simulink model "Aircraft_Model"  (R2026a)
settings: Solver=VariableStepAuto  StopTime=tEnd
values from neighbouring files (symbols this model uses):
  tEnd = 75    [Initial_Conds.m]
  U0 = [delta_ail;delta_ele;delta_rud;delta_thr]    [Initial_Conds.m]
  x0 = [x0;y0;z0;u0;v0;w0;phi0;theta0;psi0;p0;q0;r0]    [Initial_Conds.m]
undefined symbols (not defined in the file or in its folder): Non_Linear_Model_V1
libraries: aerolibanim x1
settings Model: Creator=hakka  LastModifiedBy=hakka

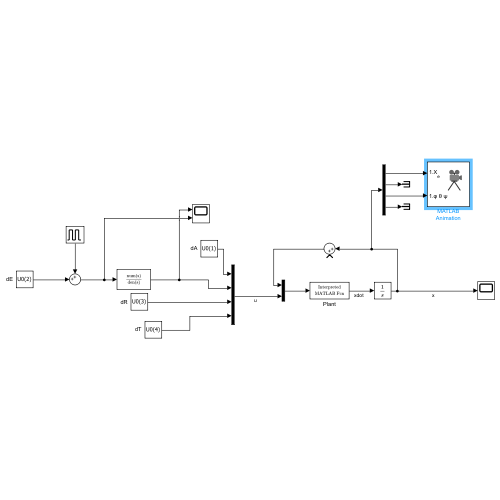
[thumbnail: Simulink's stored preview of the top-level diagram]
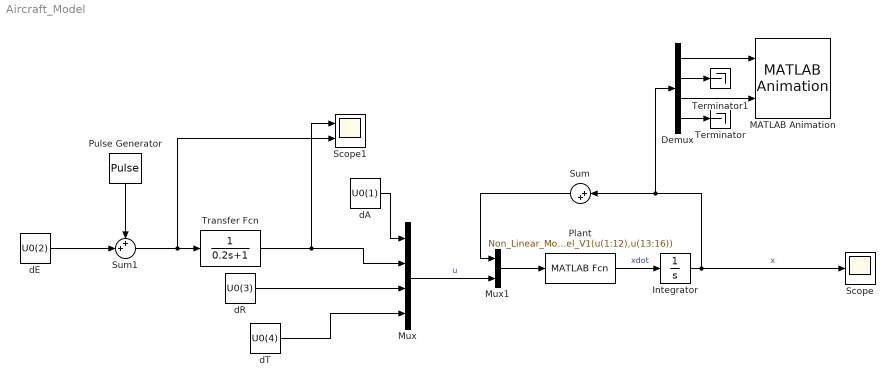
== system Aircraft_Model ==
  Demux : Demux  Outputs=[3 3 3 3]
  Integrator : Integrator  InitialCondition=x0
  MATLAB Animation : aerolibanim/MATLAB Animation  Tag=Matlab Animation 6 DOF  Vehicles=1  Geometries='pa24-250_orange.ac'  BoundingBoxCoordinates=[-100,100,-100,100,-100,100]  CameraOffset=[150,150,0]  CameraViewAngle=3  SampleTime=0.1  FigurePosition=[403,50,619,758]
  Mux : Mux
  Mux1 : Mux  Inputs=2
  Plant : MATLABFcn  MATLABFcn=Non_Linear_Model_V1(u(1:12),u(13:16))
  Pulse Generator : DiscretePulseGenerator  PulseType=Time based  Amplitude=0.05  Period=(tEnd/2)+5  PulseWidth=5  PhaseDelay=25
  Scope : Scope
      settings: ActiveDisplayYMinimum=-0.21358140820806887  ActiveDisplayYMaximum=0.10465761191012857
  Scope1 : Scope  NumInputPorts=2
      settings: ActiveDisplayYMinimum=-0.014196127760530999  ActiveDisplayYMaximum=0.048303872239469005
  Sum : Sum  Inputs=|++
  Sum1 : Sum  Inputs=++|
  Terminator : Terminator
  Terminator1 : Terminator
  Transfer Fcn : TransferFcn  Numerator=1  Denominator=[0.2 1]
  dA : Constant  Value=U0(1)
  dE : Constant  Value=U0(2)
  dR : Constant  Value=U0(3)
  dT : Constant  Value=U0(4)
  wires:
  Plant/1 -> Integrator/1  "xdot"
  Integrator/1 -> Scope/1, Demux/1, Sum/1  "x"
  dA/1 -> Mux/1
  dR/1 -> Mux/3
  dT/1 -> Mux/4
  Mux/1 -> Mux1/2  "u"
  Mux1/1 -> Plant/1
  dE/1 -> Sum1/2
  Sum/1 -> Mux1/1
  Demux/1 -> MATLAB Animation/1
  Demux/3 -> MATLAB Animation/2
  Demux/4 -> Terminator/1
  Demux/2 -> Terminator1/1
  Sum1/1 -> Scope1/2, Transfer Fcn/1
  Pulse Generator/1 -> Sum1/1
  Transfer Fcn/1 -> Mux/2, Scope1/1
